simulink model "fig3"  (R2021b)
settings: Solver=VariableStepAuto  StartTime=0.0  StopTime=10.0  RelTol=1e-3
libraries: dspfdesign x2, simulink x2
settings Model: Creator=Alex  LastModifiedBy=Alex

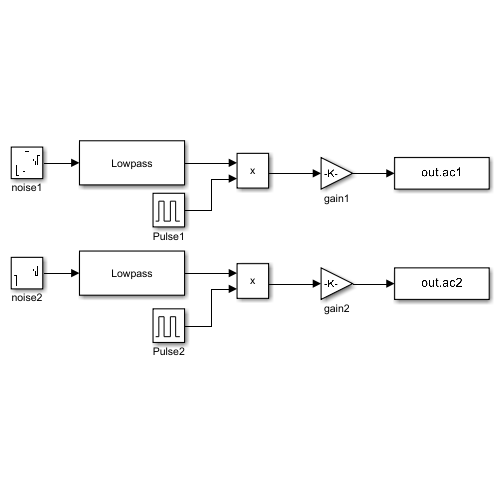
[thumbnail: Simulink's stored preview of the top-level diagram]
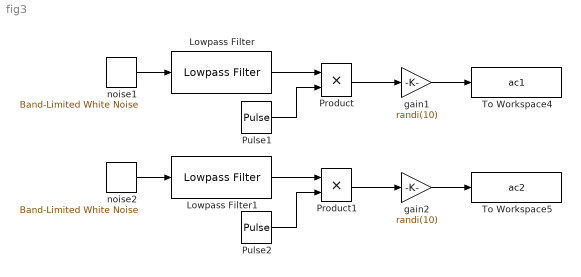
== system fig3 ==
  Lowpass Filter : dspfdesign/Lowpass Filter  FilterType=FIR  DesignForMinimumOrder=on  FilterOrder=50  PassbandFrequency=0.1  StopbandFrequency=30  PassbandRipple=0.1  StopbandAttenuation=80  InheritSampleRate=off  SampleRate=100  SimulateUsing=Interpreted execution  roundingMode=Floor  coeffsDataTypeStr=fixdt(1,16)
  Lowpass Filter1 : dspfdesign/Lowpass Filter  FilterType=FIR  DesignForMinimumOrder=on  FilterOrder=50  PassbandFrequency=0.1  StopbandFrequency=30  PassbandRipple=0.1  StopbandAttenuation=80  InheritSampleRate=off  SampleRate=100  SimulateUsing=Interpreted execution  roundingMode=Floor  coeffsDataTypeStr=fixdt(1,16)
  Product : Product
  Product1 : Product
  Pulse1 : DiscretePulseGenerator  PulseType=Time based  Period=randi(10)/10  PulseWidth=randi(9)*10  PhaseDelay=0.5
  Pulse2 : DiscretePulseGenerator  PulseType=Time based  Period=randi(10)/10  PulseWidth=randi(9)*10  PhaseDelay=0.5
  To Workspace4 : ToWorkspace  VariableName=ac1  SaveFormat=Timeseries  SampleTime=-1
      settings: Decimation=10
  To Workspace5 : ToWorkspace  VariableName=ac2  SaveFormat=Timeseries  SampleTime=-1
      settings: Decimation=10
  gain1 : Gain  Gain=randi(10)
  gain2 : Gain  Gain=randi(10)
  noise1 : simulink/Sources/Band-Limited White Noise  Cov=[0.1]  Ts=0.01  seed=randi(10000)
  noise2 : simulink/Sources/Band-Limited White Noise  Cov=[0.1]  Ts=0.01  seed=randi(10000)
  wires:
  Product1/1 -> gain2/1
  Pulse2/1 -> Product1/2
  Lowpass Filter1/1 -> Product1/1
  Product/1 -> gain1/1
  noise2/1 -> Lowpass Filter1/1
  noise1/1 -> Lowpass Filter/1
  Lowpass Filter/1 -> Product/1
  gain1/1 -> To Workspace4/1
  gain2/1 -> To Workspace5/1
  Pulse1/1 -> Product/2
